simulink model "CP_SFC_NLin_b_n9329013"  (R2017b)
settings: Solver=ode4  StartTime=0.0  StopTime=10.0  FixedStep=0.02  RelTol=1e-3
values from neighbouring files (symbols this model uses):
  g = 9.81    [CP_ContrSys_Lin_a_Mainfile_n9329013.m]    (also in CP_ContrSys_Lin_b_Mainfile_n9329013.m; MainFile_9329013.m; MainFile_Linearised_a_9329013.m; MainFile_Linearised_b_9329013.m)
  initial_cond = [0.2,20*pi/180, 0,0]'    [CP_ContrSys_Lin_a_Mainfile_n9329013.m]    (also in CP_ContrSys_Lin_b_Mainfile_n9329013.m = [0.2,200*pi/180, 0,0]')
  l = 0.2    [CP_ContrSys_Lin_a_Mainfile_n9329013.m]    (also in CP_ContrSys_Lin_b_Mainfile_n9329013.m; MainFile_9329013.m; MainFile_Linearised_a_9329013.m; MainFile_Linearised_b_9329013.m)
  m = 0.15    [CP_ContrSys_Lin_a_Mainfile_n9329013.m]    (also in CP_ContrSys_Lin_b_Mainfile_n9329013.m; MainFile_9329013.m; MainFile_Linearised_a_9329013.m; MainFile_Linearised_b_9329013.m)
  Mc = 0.4    [CP_ContrSys_Lin_a_Mainfile_n9329013.m]    (also in CP_ContrSys_Lin_b_Mainfile_n9329013.m; MainFile_9329013.m; MainFile_Linearised_a_9329013.m; MainFile_Linearised_b_9329013.m)
undefined symbols (not defined in the file or in its folder): Kb
settings Model: Creator=Koh Kim Hai  LastModifiedBy=Koh Kim Hai
settings DataIOCC: TimeSaveName=t

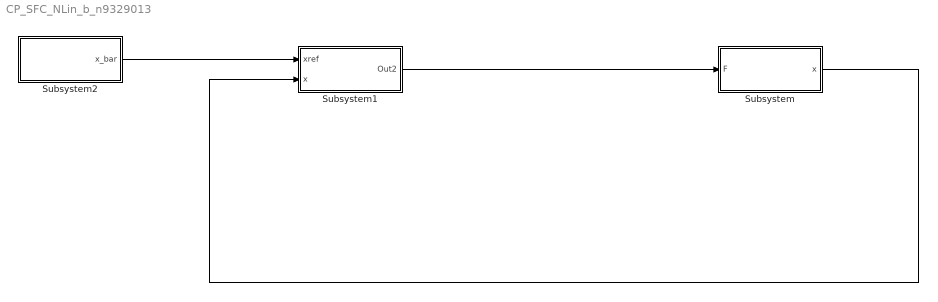
== system CP_SFC_NLin_b_n9329013 ==
  Subsystem : Subsystem
  Subsystem1 : Subsystem
  Subsystem2 : Subsystem
  wires:
  Subsystem2/1(x_bar) -> Subsystem1/1(xref)
  Subsystem1/1(Out2) -> Subsystem/1(F)
  Subsystem/1(x) -> Subsystem1/2(x)

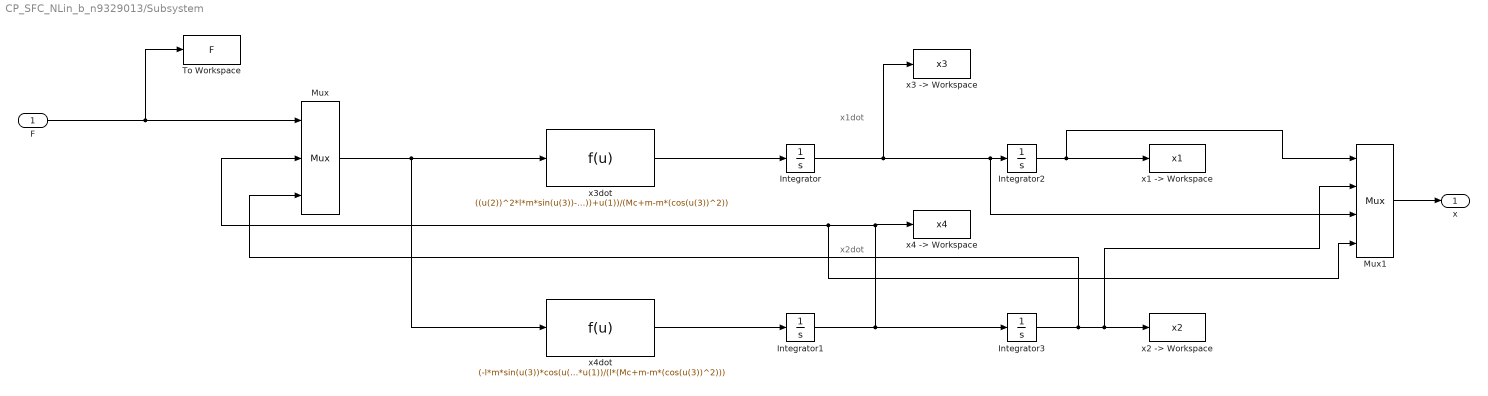
== system CP_SFC_NLin_b_n9329013/Subsystem ==
  note: x1dot
  note: x2dot
  F : Inport
  Integrator : Integrator
  Integrator1 : Integrator
  Integrator2 : Integrator  InitialCondition=initial_cond(1)
  Integrator3 : Integrator  InitialCondition=initial_cond(2)
  Mux : Mux  Inputs=3
  Mux1 : Mux
  To Workspace : ToWorkspace  VariableName=F  SampleTime=-1
  "x1 -> Workspace" : ToWorkspace  VariableName=x1  SampleTime=-1
  "x2 -> Workspace" : ToWorkspace  VariableName=x2  SampleTime=-1
  "x3 -> Workspace" : ToWorkspace  VariableName=x3  SampleTime=-1
  x3dot : Fcn  Expr=((u(2))^2*l*m*sin(u(3))-g*m*sin(u(3))*cos(u(3))+u(1))/(Mc+m-m*(cos(u(3))^2))
  "x4 -> Workspace" : ToWorkspace  VariableName=x4  SampleTime=-1
  x4dot : Fcn  Expr=(-l*m*sin(u(3))*cos(u(3))*(u(2))^2+g*(Mc+m)*sin(u(3))-cos(u(3))*u(1))/(l*(Mc+m-m*(cos(u(3))^2)))
  x : Outport
  wires:
  Integrator3/1 -> Mux/3, Mux1/2, "x2 -> Workspace"/1
  Integrator/1 -> "x3 -> Workspace"/1, Mux1/3, Integrator2/1
  F/1 -> To Workspace/1, Mux/1
  Integrator1/1 -> Mux1/4, Mux/2, "x4 -> Workspace"/1, Integrator3/1
  Mux/1 -> x4dot/1, x3dot/1
  Integrator2/1 -> Mux1/1, "x1 -> Workspace"/1
  x3dot/1 -> Integrator/1
  x4dot/1 -> Integrator1/1
  Mux1/1 -> x/1

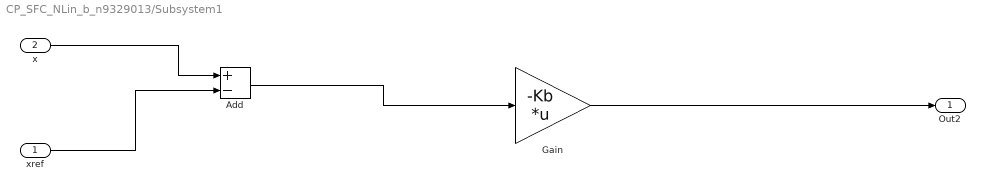
== system CP_SFC_NLin_b_n9329013/Subsystem1 ==
  xref : Inport
  x : Inport  Port=2
  Add : Sum  Inputs=+-
  Gain : Gain  Gain=-Kb  Multiplication=Matrix(K*u)
  Out2 : Outport
  wires:
  Gain/1 -> Out2/1
  xref/1 -> Add/2
  x/1 -> Add/1
  Add/1 -> Gain/1

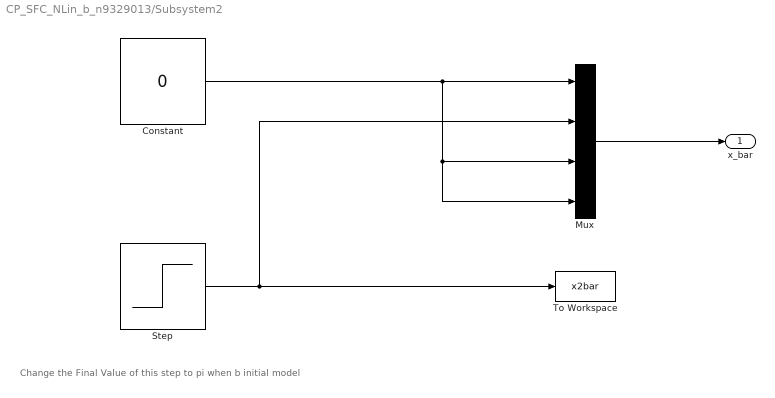
== system CP_SFC_NLin_b_n9329013/Subsystem2 ==
  note: Change the Final Value of this step to pi when b initial model
  Constant : Constant  Value=0
  Mux : Mux
  Step : Step  Time=0  After=pi  SampleTime=0
  To Workspace : ToWorkspace  VariableName=x2bar  SampleTime=-1
  x_bar : Outport
  wires:
  Mux/1 -> x_bar/1
  Constant/1 -> Mux/4, Mux/3, Mux/1
  Step/1 -> To Workspace/1, Mux/2
